simulink model "testCerebusParseInC"  (R2015a)
settings: Solver=FixedStepDiscrete  StartTime=0.0  StopTime=Inf  FixedStep=0.001  RelTol=1e-3
undefined symbols (not defined in the file or in its folder): gcbh, macaddr, mxpcnbunlink, mxpcnetworkconfig, mxpcrtudprx
libraries: slrtlib x4, dspindex x2, xpcnetworkbufferlib x2, xpciplib x2, simulink x1, xpcethernetlib x1, commfilt2 x1
settings Model: xpc_rtwmakecfg_data=_xpciplib__xpcnblib__xpcetherlib__xpcether8255xlib__xpcetherGbElib_  SimulationMode=external  Creator=djoshea  LastModifiedBy=shenoylab
settings SolverCC: EnableConcurrentExecution=on
settings OptimizationCC: BlockReduction=off  OptimizeBlockIOStorage=off  BufferReuse=off  GlobalBufferReuse=off  ExpressionFolding=off  LocalBlockOutputs=off  SimCompilerOptimization=on
settings HardwareCC: ProdIntDivRoundTo=Zero  ProdEndianess=LittleEndian  ProdLongLongMode=on  ProdHWDeviceType=Generic->32-bit x86 compatible  TargetBitPerLong=64  TargetBitPerPointer=64  TargetIntDivRoundTo=Zero  TargetEndianess=LittleEndian  TargetWordSize=64  TargetHWDeviceType=Intel->x86-64
settings SFSimCC: SimBuildMode=sf_nonincremental_build
settings RTWCC: SystemTargetFile=slrt.tlc  TemplateMakefile=slrt_default_tmf  Description=Simulink Real-Time  GenerateReport=on  CustomSource=cerebusParse.c  LaunchReport=on  RTWCompilerOptimization=on
settings CodeAppCC: MaxIdLength=95  MATLABSourceComments=on
settings SimulinkRealTimeCC: GeneratePreprocessorConditionals=Disable all

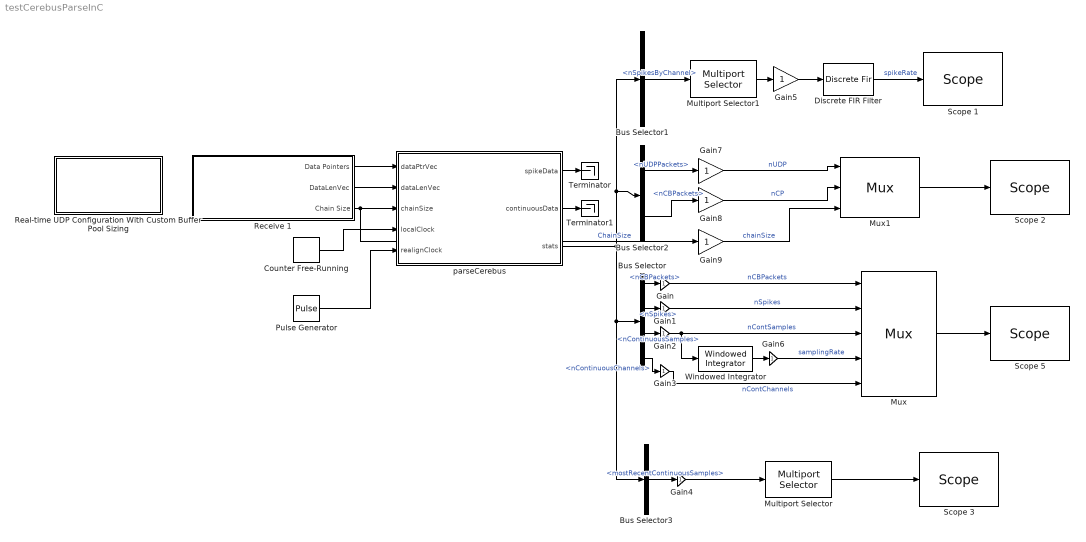
== system testCerebusParseInC ==
  Bus Selector : BusSelector  OutputSignals=nCBPackets,nSpikes,nContinuousSamples,nContinuousChannels
  Bus Selector1 : BusSelector  OutputSignals=nSpikesByChannel
  Bus Selector2 : BusSelector  OutputSignals=nUDPPackets,nCBPackets
  Bus Selector3 : BusSelector  OutputSignals=mostRecentContinuousSamples
  Counter Free-Running : simulink/Sources/Counter Free-Running  NumBits=32  tsamp=0.001
  Discrete FIR Filter : DiscreteFir  Coefficients=exp(-(0:100)/20)
  Gain{,1..9} (10 alike) : Gain  OutDataTypeStr=double
  Multiport Selector : dspindex/Multiport Selector  rowsOrCols=Rows  idxCellArray={ 1 : 10 }  idxErrMode=Clip Index
  Multiport Selector1 : dspindex/Multiport Selector  rowsOrCols=Rows  idxCellArray={ 1 : 10 }  idxErrMode=Clip Index
  Mux : Mux  Inputs=5
      settings: DisplayOption=signals
  Mux1 : Mux  Inputs=3
      settings: DisplayOption=signals
  Pulse Generator : DiscretePulseGenerator  Period=100000  PhaseDelay=20  SampleTime=0.001
  Real-time UDP Configuration With Custom Buffer Pool Sizing : Subsystem  InitFcn=mxpcnetworkconfig(1);  mask(xpcnwconfig){ID=1, IpAddress=192.168.137.4, SubnetMask=255.255.255.0, Gateway=0.0.0.0, EthDrv=Intel 8255x, PciBus=4, PciSlot=4, udpID=0, PoolSizes=[8196 512 4096 65535]}
      mask prompts: ID "Device ID:"; IpAddress "IP Address:"; SubnetMask "Subnet Mask:"; EthDrv "Ethernet Driver:"; PciBus "PCI Bus:"; PciSlot "PCI Slot:"; udpID "Internal UDP ID:"; PoolSizes "Buffer pool sizes (256, 512, 1024, 2048):"
      mask help: Configure network interface for real-time UDP communication.
      mask init:
      | IpAddress = ipaddr(IpAddress);
      | SubnetMask = ipaddr(SubnetMask);
      | Gateway = ipaddr(Gateway);
      | udpID = ID - 1;
      | 
      | [MaskDisplay] = mxpcnetworkconfig(2, ID, EthDrv, PciBus, PciSlot);
      | set_param(gcb, 'MaskDisplay', MaskDisplay);
      mask Help: eval('xpcdoc(''RT_NETWORK_CONFIGURATION'')');
      mask TypeOptions ID: Ethernet Init /ID
      mask TypeOptions EthDrv: Ethernet Init /Driver
      mask TypeOptions PoolSizes: Buffer Mngmt /PoolSizes
      mask Display: disp('Real-time UDP\nConfiguration\nBus: 4 Slot: 4\nId: 1\nIntel 8255x');
  Receive 1 : Subsystem  InitFcn=mxpcrtudprx(1, get_param(gcbh, 'ID'));  mask(rtudpreceive){ID=1, Receive1=0.0.0.0, Receive2=1002, maxPackets=1000, Receive4=0.001, udpID=0}
      mask prompts: ID "Device ID:"; Receive1 "Source IP Address:"; Receive2 "Local (destination) port:"; maxPackets "Max Packets"; Receive4 "Sample time:"; udpID "Internal UDP ID:"
      mask help:
      | Receive data over UDP network on a dedicated network interface.
      |
      | This block receives data on the specified local (destination) port. To receive all data sent to this port, set 'Source IP Address' to 0.0.0.0. To receive data sent to this port from a specific remote source, enter the IP address of that source.
      mask init:
      | Receive1 = ipaddr(Receive1);
      | udpID = ID -1;
      mask Help: eval('xpcdoc(''RT_UDP_RECEIVE'')');
      mask TypeOptions ID: 1 | 2 | 3 | 4 | 5 | 6 | 7 | 8
      mask Display:
      | disp('UDP Expose\nId: 1');
      | port_label('output', 1, 'DataPtrVec');
      | port_label('output', 2, 'DataLenVec');
      | port_label('output', 3, 'Chain Size');
  Scope 1 : slrtlib/Displays and Logging/Scope   scopeno=1  scopetype=Target  autostart=on  viewmode=Graphical rolling  formatstr='%5.0f,%5.0f'  grid=on  ylimits=[0 5]  nosamples=1000  noprepostsamples=0  interleave=1  triggermode=FreeRun  triggersignal=1  trigsignalfromport=off  triggerlevel=0.0  triggerslope=Either  triggerscope=1  triggersample=0  filename=data.dat  mode=Lazy  writesize=512  autorestart=off  dynamicfilemode=off  maxwritefilesize=512*1024^2
  Scope 2 : slrtlib/Displays and Logging/Scope   scopeno=2  scopetype=Target  autostart=on  viewmode=Graphical rolling  formatstr='%5.0f,%5.0f'  grid=on  ylimits=[0 50]  nosamples=1000  noprepostsamples=0  interleave=1  triggermode=FreeRun  triggersignal=1  trigsignalfromport=off  triggerlevel=0.0  triggerslope=Either  triggerscope=1  triggersample=0  filename=data.dat  mode=Lazy  writesize=512  autorestart=off  dynamicfilemode=off  maxwritefilesize=512*1024^2
  Scope 3 : slrtlib/Displays and Logging/Scope   scopeno=3  scopetype=Target  autostart=on  viewmode=Graphical rolling  formatstr='%5.0f,%5.0f,%5.0f,%5.0f'  grid=on  ylimits=[0 0]  nosamples=1000  noprepostsamples=0  interleave=1  triggermode=FreeRun  triggersignal=1  trigsignalfromport=off  triggerlevel=0.0  triggerslope=Either  triggerscope=1  triggersample=0  filename=data.dat  mode=Lazy  writesize=512  autorestart=off  dynamicfilemode=off  maxwritefilesize=512*1024^2
  Scope 5 : slrtlib/Displays and Logging/Scope   scopeno=6  scopetype=Target  autostart=on  viewmode=Numerical  formatstr='%5.0f,%5.0f,%5.0f,%5.0f,%5.0f'  grid=on  ylimits=[0 0]  nosamples=1000  noprepostsamples=0  interleave=1  triggermode=FreeRun  triggersignal=1  trigsignalfromport=off  triggerlevel=0.0  triggerslope=Either  triggerscope=1  triggersample=0  filename=data.dat  mode=Lazy  writesize=512  autorestart=off  dynamicfilemode=off  maxwritefilesize=512*1024^2
  Terminator : Terminator
  Terminator1 : Terminator
  Windowed Integrator : commfilt2/Windowed Integrator  integperiod=1000  roundingMode=Floor  overflowMode=off  InputProcessing=Columns as channels (frame based)
  parseCerebus : MATLAB Function  TreatAsAtomicUnit=on
  wires:
  Mux/1 -> Scope 5/1
  Receive 1/1(Data Pointers) -> parseCerebus/1(dataPtrVec)
  Receive 1/2(DataLenVec) -> parseCerebus/2(dataLenVec)
  Receive 1/3(Chain Size) -> Gain9/1, parseCerebus/3(chainSize)  "ChainSize"
  Counter Free-Running/1 -> parseCerebus/4(localClock)
  Pulse Generator/1 -> parseCerebus/5(realignClock)
  parseCerebus/3(stats) -> Bus Selector1/1, Bus Selector2/1, Bus Selector3/1, Bus Selector/1
  Bus Selector/1 -> Gain/1  "<nCBPackets>"
  Bus Selector/2 -> Gain1/1  "<nSpikes>"
  Bus Selector/3 -> Gain2/1  "<nContinuousSamples>"
  Gain/1 -> Mux/1  "nCBPackets"
  Gain1/1 -> Mux/2  "nSpikes"
  Gain2/1 -> Windowed Integrator/1, Mux/3  "nContSamples"
  Bus Selector/4 -> Gain3/1  "<nContinuousChannels>"
  Gain3/1 -> Mux/5  "nContChannels"
  Bus Selector3/1 -> Gain4/1  "<mostRecentContinuousSamples>"
  Gain4/1 -> Multiport Selector/1
  Multiport Selector/1 -> Scope 3/1
  Windowed Integrator/1 -> Gain6/1
  Bus Selector1/1 -> Multiport Selector1/1  "<nSpikesByChannel>"
  Multiport Selector1/1 -> Gain5/1
  Discrete FIR Filter/1 -> Scope 1/1  "spikeRate"
  Gain5/1 -> Discrete FIR Filter/1
  parseCerebus/1(spikeData) -> Terminator/1
  Gain6/1 -> Mux/4  "samplingRate"
  parseCerebus/2(continuousData) -> Terminator1/1
  Bus Selector2/1 -> Gain7/1  "<nUDPPackets>"
  Bus Selector2/2 -> Gain8/1  "<nCBPackets>"
  Gain7/1 -> Mux1/1  "nUDP"
  Gain8/1 -> Mux1/2  "nCP"
  Mux1/1 -> Scope 2/1
  Gain9/1 -> Mux1/3  "chainSize"

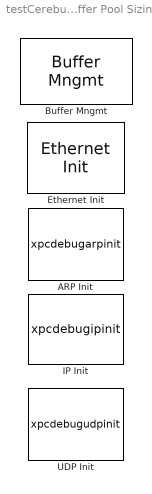
== system testCerebusParseInC/Real-time UDP Configuration With Custom Buffer Pool Sizing ==
  "ARP Init " : S-Function  Priority=0  FunctionName=xpcdebugarpinit  Parameters=Stats, Interface, IpAddress, SubnetMask, Gateway, EthernetId, Flags, BlockId, Retry, Timeout, Expiration, StaticAddressListIp, StaticAddressListMac, DiscoveryList, MulticastList, SampleTime  mask(arpinit){Interface=udpID, IpAddress=IpAddress, SubnetMask=SubnetMask, Gateway=Gateway, EthernetId=ID, BlockId=0, SampleTime=-1, Flags=hex2dec('00000697'), Stats=off, Retry=5, Timeout=20, Expiration=20*60, StaticAddressListIp=[], StaticAddressListMac=[], DiscoveryList=[], MulticastList=[]}
      mask prompts: IpAddress "IP Address"; SubnetMask "Subnet Mask"; EthernetId "Ethernet ID"; BlockId "Block ID"; SampleTime "Sample Time"; Stats "Statistics Port"; StaticAddressListIp "[Static IP]"; StaticAddressListMac "[Static MAC]"; DiscoveryList "[Discovery IP]"; MulticastList "[Multicast IP]"
      mask help: ARP Init
      mask init:
      | xpclinklib('xpciplib');
      mask Help: web('arpdebug.htm',  '-helpbrowser');
      mask Display: disp('ARP Init');
  "Buffer Mngmt " : xpcnetworkbufferlib/Buffer Mngmt   Priority=-1  SampleTime=-1  PoolSizes=PoolSizes  ShowTune=off
  "Ethernet Init " : xpcethernetlib/Ethernet Init   Priority=-1  ID=1  Driver=Intel 8255x  Bus=PciBus  Slot=PciSlot  SampleTime=-1  AddressSource=EEPROM  MAC=macaddr('00:00:00:00:00:00')  TxSA=off  RxPromiscuous=off  Multicast={}  RxBad=off  RxShort=off  MaxMTU=1518  TxThreshold=224  TxBuffers=128  RxBuffers=64  ShowTune=off  NumRxBlks=1
  "IP Init " : S-Function  Priority=1  FunctionName=xpcdebugipinit  Parameters=Stats, Group, ArpId, IpAddress, SubnetMask, DefaultGateway, DefaultInterface, Flags, ToS, StartingId, TTL, SampleTime  mask(ipinit){Group=udpID, ArpId=[udpID], IpAddress=[IpAddress], SubnetMask=[SubnetMask], DefaultGateway=Gateway, DefaultInterface=0, SampleTime=-1, Flags=hex2dec('00000005'), ToS=hex2dec('00'), StartingId=10000, TTL=64, Stats=off}
      mask prompts: ArpId "[ARP ID]"; IpAddress "[IP Address]"; SubnetMask "[Subnet Mask]"; DefaultGateway "Default Gateway"; DefaultInterface "Default Interface"; SampleTime "Sample Time"; StartingId "Starting Id"; Stats "Statistics Port"
      mask help: IP Init
      mask init:
      | xpclinklib('xpciplib');
      mask Help: web('ipdebug.htm',  '-helpbrowser');
      mask Display: disp('IP Init');
  "UDP Init " : S-Function  Priority=2  FunctionName=xpcdebugudpinit  Parameters=Stats, Group, StartingPort, Flags, SampleTime  mask(udpinit){Group=udpID, StartingPort=10000, Flags=hex2dec('00000001'), SampleTime=-1, Stats=off}
      mask prompts: StartingPort "Starting Port"; SampleTime "Sample Time"; Stats "Statistics Port"
      mask help: UDP Init
      mask init:
      | xpclinklib('xpciplib');
      mask Help: web('udpdebug.htm',  '-helpbrowser');
      mask Display: disp('UDP Init');

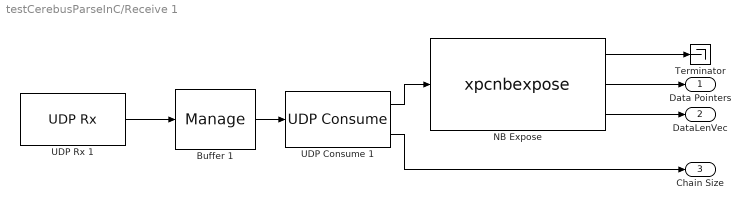
== system testCerebusParseInC/Receive 1 ==
  Buffer 1 : xpcnetworkbufferlib/Manage   ChainSize=maxPackets  BufferSize=maxPackets*5  Threshold=0
  NB Expose : S-Function  InitFcn=mxpcnbunlink(1,0);  FunctionName=xpcnbexpose  Parameters=vectorLength  mask(xpcnbunlink){VectorLength=maxPackets}
      mask prompts: VectorLength "Vector length (-1 inherit):"
      mask help: Unlink a chain into a vector of network buffers.
      mask init:
      | [vectorLength] = mxpcnbunlink(2, VectorLength);
      mask Help: eval('xpcdoc(''NB_Unlink'')');
      mask Display:
      | disp('NB Expose');
      | port_label('output', 1, 'NBVec');
      | port_label('output', 2, 'DataPtrVec');
      | port_label('output', 3, 'DataLenVec');
  Terminator : Terminator
  UDP Consume 1 : xpciplib/UDP Consume   Group=udpID  VectorSize=0  SampleTime=Receive4
  UDP Rx 1 : xpciplib/UDP Rx   Priority=5  Group=udpID  sip=Any  SourceAddress=Receive1  lup=Specify  LocalPort=Receive2  SampleTime=Receive4
  Data Pointers : Outport
  DataLenVec : Outport  Port=2
  Chain Size : Outport  Port=3
  wires:
  UDP Consume 1/1 -> NB Expose/1
  Buffer 1/1 -> UDP Consume 1/1
  UDP Rx 1/1 -> Buffer 1/1
  UDP Consume 1/2 -> Chain Size/1
  NB Expose/1 -> Terminator/1
  NB Expose/2 -> Data Pointers/1
  NB Expose/3 -> DataLenVec/1

== matlab function testCerebusParseInC/parseCerebus ==
  data: dataPtrVec input uint32; dataLenVec input uint32; chainSize input size=1; spikeData output Bus: SpikeDataBus size=1; continuousData output Bus: ContinuousDataBus size=1; stats output Bus: CerebusStatisticsBus size=1; localClock input uint32 size=1; realignClock input size=1; CerebusInfo parameter size=1
function [spikeData, continuousData, stats] = parseCerebus(dataPtrVec, dataLenVec, chainSize, localClock, realignClock, CerebusInfo)
%#codegen

% these pointers are coder.opaque, they will be used only via ceval calls
% within CerebusParse
% [pp, pBufferEnd] = CerebusParse.nbExtractPacketData(nb);

% length of a spike cbPKT in the lab (96 bytes for the waveform, 4 bytes for
% the min and max in the waveform, 12 bytes for spike sorting details
% giving a total of 112 bytes

    % for aligning cerebus clock (30 kHz) to local clock (1 kHz) at start of each trial
    persistent pCerebusClockReference;
    persistent pCerebusClockRecent;
    persistent pLocalClockReference;
    if isempty(pCerebusClockReference)
        pCerebusClockReference = single(NaN);
        pLocalClockReference = single(NaN);
        pCerebusClockRecent = uint32(0);
    end 

    cb_time = uint32(0);
    msOffset = single(0);

    % build the SpikeDataBus fields as full-size copies here
    spikeTimeOffsets = zeros([CerebusInfo.MaxSpikesPerTick 1], 'single');
    spikeChannels = zeros([CerebusInfo.MaxSpikesPerTick 1], 'uint8');
    spikeUnits = zeros([CerebusInfo.MaxSpikesPerTick 1], 'uint8');
    spikeWaveforms = zeros([CerebusInfo.WaveformNumSamples CerebusInfo.MaxSpikesPerTick], 'int16');
    
    % build the ContinuousDataBus fields as full-size copies here
    continuousTimeOffsets = zeros([CerebusInfo.MaxChannels 1], 'single');
    continuousSamples = zeros([CerebusInfo.MaxChannels CerebusInfo.MaxContinuousSamplesPerTick], 'int16');
    
    stats = initializeBus_CerebusStatisticsBus();
    stats.nSpikes = uint32(0);
    stats.nContinuousChannels = uint16(0);
    stats.nContinuousSamples = uint32(0);
    stats.nCBPackets = uint32(0);

    for iP = uint32(1):uint32(chainSize)
        if dataPtrVec(iP) == 0 || dataLenVec(iP) == 0
            continue;
        end

        stats.nUDPPackets = stats.nUDPPackets + uint32(1);
        stats.nUDPBytes = stats.nUDPBytes + uint32(dataLenVec(iP));
        
        [pp, pBufferEnd] = CerebusParse.getPointersFromDataPtr(dataPtrVec(iP), dataLenVec(iP));
        stats.nCBPackets = stats.nCBPackets + uint32(1);

        while true
            cb_time = CerebusParse.getTime(pp);

            if CerebusParse.isSpikePacket(pp)
                % Received spike packet
                if stats.nSpikes < uint32(CerebusInfo.MaxSpikesPerTick)
                    stats.nSpikes = stats.nSpikes + uint32(1);

                    cb_channel = CerebusParse.getChannel(pp);
                    cb_unit = CerebusParse.getSpikeUnit(pp);

                    if cb_channel >= 1 && cb_channel <= CerebusInfo.MaxChannels
                       msOffset = CerebusParse.computeTimeOffsetMs(cb_time, localClock, ...
                           pLocalClockReference, pCerebusClockReference);

                        % store spike info and waveform
                        spikeTimeOffsets(stats.nSpikes) = msOffset;
                        spikeChannels(stats.nSpikes) = cb_channel;
                        spikeUnits(stats.nSpikes) = cb_unit;
                        
                        % copy spike waveform directly into waveforms matrix
                        spikeWaveforms = CerebusParse.copyContinuousSamplesToBufferColumn(pp, spikeWaveforms, stats.nSpikes);
                        
                        % update statistics
                        stats.nSpikesByChannel(cb_channel) = stats.nSpikesByChannel(cb_channel) + uint32(1);
                    end
                end

            elseif CerebusParse.isContinuousPacketForGroup(pp, uint8(CerebusInfo.ContinuousGroupId))
                % receieved continuous data sample for the appropriate group id
                if stats.nContinuousSamples < uint32(CerebusInfo.MaxContinuousSamplesPerTick)
                    stats.nContinuousSamples = stats.nContinuousSamples + uint32(1);

                    msOffset = CerebusParse.computeTimeOffsetMs(cb_time, localClock, ...
                           pLocalClockReference, pCerebusClockReference);

                    continuousTimeOffsets(stats.nContinuousSamples) = msOffset;

                    if stats.nContinuousChannels == uint16(0)
                        % because the number of continuous channels is not known ahead of time,
                        % declare the size of continuousData now that we
                        % have a non-zero channel count
                        stats.nContinuousChannels = uint16(min(CerebusInfo.MaxChannels, CerebusParse.getContinuousNumChannels(pp)));
                    end
                    
                    % copy in the samples
                    continuousSamples = CerebusParse.copyContinuousSamplesToBufferColumn(pp, continuousSamples, stats.nContinuousSamples);
                end
            end

            % jump to the next cbPKT
            if ~CerebusParse.hasNext(pp, pBufferEnd)
                break;
            end
            pp = CerebusParse.getNext(pp);
            stats.nCBPackets = stats.nCBPackets + uint32(1);
        end
    end
    
    % build SpikeDataBus
    spikeData.spikeTimeOffsets = spikeTimeOffsets(1:stats.nSpikes);
    spikeData.spikeChannels = spikeChannels(1:stats.nSpikes);
    spikeData.spikeUnits = spikeUnits(1:stats.nSpikes);
    spikeData.spikeWaveforms = spikeWaveforms(:, 1:stats.nSpikes);

    % build ContinuousDataBus
    continuousData.continuousTimeOffsets = continuousTimeOffsets(1:stats.nContinuousSamples);
    continuousData.continuousData = continuousSamples(1:stats.nContinuousChannels, 1:stats.nContinuousSamples);
    
    if cb_time > uint32(0)
        pCerebusClockRecent = cb_time;
    end
    stats.cerebusClock = pCerebusClockRecent;
    stats.clockOffset = msOffset;

    % store the most recent continuous sample in the stats
    if size(continuousData.continuousData, 2) > 0
        stats.mostRecentContinuousSamples(1:stats.nContinuousChannels) = continuousData.continuousData(1:stats.nContinuousChannels, 1);
    end

    % reset the clock alignment after the buffer has been flushed of old packets
    % and if starting a new trial
    if cb_time > 0 && localClock > 10 && (isnan(pCerebusClockReference) || realignClock)
        % reset the clock alignment between local (1 kHz) and Cerebus (30 kHz)
        % typically at the end of trials
        pCerebusClockReference = single(cb_time);
        pLocalClockReference = single(localClock);
        %coder.ceval('printf', [char('Cerebus align cc %g, lc %g') 10 0], pCerebusClockReference, pLocalClockReference);
    end

end
